simulink model "prob2_214869"  (R2020a)
settings: Solver=VariableStepAuto  StartTime=0.0  StopTime=100.0  RelTol=1e-3
undefined symbols (not defined in the file): sigbuilder_block
settings Model: Creator=sonal  LastModifiedBy=sonal

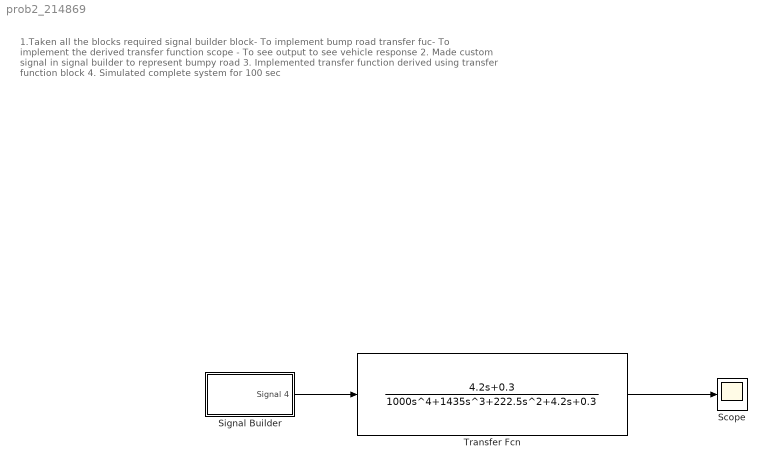
== system prob2_214869 ==
  note: 1.Taken all the blocks required
      | signal builder block- To implement bump road
      | transfer fuc- To implement the derived transfer function
      | scope - To see output to see vehicle response
      |
      | 2. Made custom signal in signal builder to represent bumpy road
      |
      | 3. Implemented transfer function derived using transfer function block
      |
      | 4. Simulated complete system for 100 sec
  Scope : Scope
  Signal Builder : Subsystem  Tag=STV Subsys  LoadFcn=sigbuilder_block('load');  StartFcn=sigbuilder_block('start');  StopFcn=sigbuilder_block('stop');  ClipboardFcn=sigbuilder_block('clipboard');  mask(Sigbuilder block){tuvar=[0:10]}
      mask help: Simulink:masks:SigbuilderBlock_MD
      mask init:
      | if ~strcmp(get_param(bdroot(gcbh),'SimulationStatus'),'stopped') tuvar = sigbuilder_block('maskInit'); end
      settings: CopyFcn=sigbuilder_block('copy');  DeleteFcn=sigbuilder_block('delete');  ModelCloseFcn=sigbuilder_block('modelClose');  PreSaveFcn=sigbuilder_block('preSave');  PauseFcn=sigbuilder_block('pause');  ContinueFcn=sigbuilder_block('continue');  NameChangeFcn=sigbuilder_block('namechange');  OpenFcn=sigbuilder_block('open',[0 30 1024.5 488.25 ]);  CloseFcn=sigbuilder_block('close');
      mask Display: plot(0, 0, 100, 100,[2, 2, 32, 32, 2], [68, 8, 8, 68, 68],[32, 2], [38, 38], [32, 19, 2],[53, 60, 44], [32, 17, 17, 2],[16, 16, 31, 31]);txt = getActiveGroup(gcbh);text(2, 100, txt,'verticalAlignment', 'top');
  Transfer Fcn : TransferFcn  Numerator=[4.2 0.3]  Denominator=[1000 1435 222.5 4.2 0.3]
  wires:
  Signal Builder/1(Signal 4) -> Transfer Fcn/1
  Transfer Fcn/1 -> Scope/1

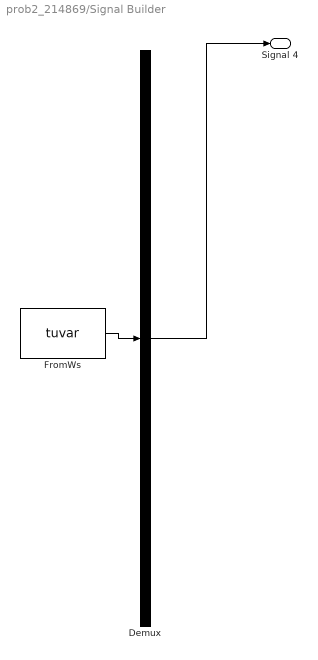
== system prob2_214869/Signal Builder ==
  Demux : Demux  Tag=STV Demux  Outputs=1
      settings: DisplayOption=none
  FromWs : FromWorkspace  Tag=STV FromWs  VariableName=tuvar
      SigBuilderData=|
      | common.afterFinalStr = 'Extrapolate'
      | common.sampleTime = 0
      | dataSet.timeRange = [0 10]
      | dataSet.name = 'Group 1'
      | sbobj.Groups.Name = 'Group 1'
      | sbobj.Groups.Signals.Name = 'Signal 4'
      | sbobj.Groups.Signals.XData = [0 0.222222222222 0.444444444444 0.666666666667 0.888888888889 1.11111111111 1.11111111111 1.33333333333 1.33333333333 1.55555555556 1.77777777778 1.77777777778 2 2 2.22222222222 2.22222222222 2.44444444444 2.44444444444 2.66666666667 2.88888888889 3.11111111111 3.11111111111 3.33333333333 3.33333333333 3.55555555556 3.55555555556 3.77777777778 3.77777777778 4 4 4.22222222222 4.22222222222 4.44444444444 4.44444444444 4.66666666667 4.88888888889 5.11111111111 5.11111111111 5.33333333333 5.33333333333 5.55555555556 5.55555555556 5.77777777778 5.77777777778 6 6 6.22222222222 6.44444444444 6.66666666667 6.88888888889 6.88888888889 7.11111111111 7.11111111111 7.33333333333 7.55555555556 7.77777777778 8 8.22222222222 8.44444444444 8.66666666667 8.88888888889 9.11111111111 9.33333333333 9.55555555556 9.77777777778 10]
      | sbobj.Groups.Signals.YData = [1 4.21393804843 5.92403876506 5.33012701892 2.71010071663 -0.710100716628 -0.5 -1 -0.9 -1.4 0.3 0.2 1 0.6 1.7 1.5 3.2 3.4 2.9 2.71010071663 -0.710100716628 0.1 -1.6 -1.3 -1.9 -1.6 0.1 0.2 -0.3 -0.6 2.6 2.5 3.6 3.5 3.9 2.71010071663 2.1 2.2 -0.4 0.3 -0.2 -0.8 0.9 0.2 0.9 1 4.21393804843 5.92403876506 5.33012701892 5.6 5.7 5.2 5.1 4 3.4 2.5 2.9 4.21393804843 5.92403876506 5.33012701892 2.71010071663 -0.710100716628 -3.33012701892 -3.92403876506 -2.21393804843 1]
  Signal 4 : Outport  Tag=STV Outport
  wires:
  FromWs/1 -> Demux/1
  Demux/1 -> Signal 4/1
